simulink library "InputDeviceHandler"  (R2016b)
settings: Solver=VariableStepAuto  StartTime=0.0  StopTime=10.0  RelTol=1e-3
settings Model: Creator=Nathan  LastModifiedBy=march

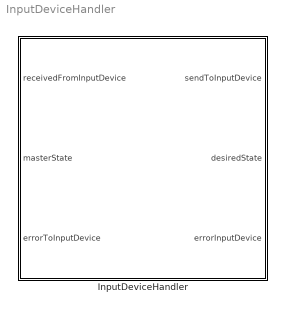
== system InputDeviceHandler ==
  InputDeviceHandler : Subsystem

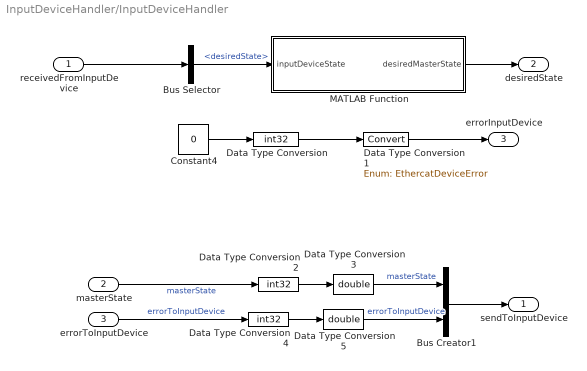
== system InputDeviceHandler/InputDeviceHandler ==
  receivedFromInputDevice : Inport  OutDataTypeStr=Bus: EtherCATReceivedFromInputDevice  BusOutputAsStruct=on
  masterState : Inport  Port=2  OutDataTypeStr=Enum: ExoskeletonState
  errorToInputDevice : Inport  Port=3
  Bus Creator1 : BusCreator  Inputs=2  OutDataTypeStr=Bus: EtherCATSendToInputDevice  NonVirtualBus=on
  Bus Selector : BusSelector  OutputSignals=desiredState
  Constant4 : Constant  Value=0
      settings: OpenFcn=|
      | b = get_param(gcb,'value');
      | if (strcmp(b,'72')),
      |   set_param (gcb,'value','0');
      | else
      |   set_param(gcb,'value','72');
      | end;
  Data Type Conversion : DataTypeConversion  OutDataTypeStr=int32
  Data Type Conversion1 : DataTypeConversion  OutDataTypeStr=Enum: EthercatDeviceError
  Data Type Conversion2 : DataTypeConversion  OutDataTypeStr=int32
  Data Type Conversion3 : DataTypeConversion  OutDataTypeStr=double
  Data Type Conversion4 : DataTypeConversion  OutDataTypeStr=int32
  Data Type Conversion5 : DataTypeConversion  OutDataTypeStr=double
  MATLAB Function : MATLAB Function  TreatAsAtomicUnit=on
  sendToInputDevice : Outport  OutDataTypeStr=Bus: EtherCATSendToInputDevice  BusOutputAsStruct=on
  desiredState : Outport  Port=2
  errorInputDevice : Outport  Port=3  OutDataTypeStr=Enum: EthercatDeviceError
  wires:
  Data Type Conversion5/1 -> Bus Creator1/2  "errorToInputDevice"
  errorToInputDevice/1 -> Data Type Conversion4/1  "errorToInputDevice"
  Data Type Conversion4/1 -> Data Type Conversion5/1
  Data Type Conversion3/1 -> Bus Creator1/1  "masterState"
  Data Type Conversion2/1 -> Data Type Conversion3/1
  MATLAB Function/1(desiredMasterState) -> desiredState/1
  Bus Selector/1 -> MATLAB Function/1(inputDeviceState)  "<desiredState>"
  receivedFromInputDevice/1 -> Bus Selector/1
  Data Type Conversion1/1 -> errorInputDevice/1
  Data Type Conversion/1 -> Data Type Conversion1/1
  masterState/1 -> Data Type Conversion2/1  "masterState"
  Bus Creator1/1 -> sendToInputDevice/1
  Constant4/1 -> Data Type Conversion/1

== matlab function InputDeviceHandler/MATLAB Function ==
  data: inputDeviceState input; desiredMasterState output
function desiredMasterState = getDesiredMasterState(inputDeviceState)
%% Translates received inputDeviceState to desired ExoskeletonState
% Copy of input device source code:
%#define SIT 0
%#define STAND 1
%#define WALK 2
%#define STONES 3
%#define STAIRS_UP 4
%#define STAIRS_DOWN 5
%#define SLOPE_UP 6
%#define SLOPE_DOWN 7
%#define MANUAL 8
switch(inputDeviceState)
    case 0 %% on disconnect, this will be zero. Need to change the values in inputDevice source
        desiredMasterState = ExoskeletonState.SITTINGDOWN;
    case 1
        desiredMasterState = ExoskeletonState.STANDINGUP;
    case 2
        desiredMasterState = ExoskeletonState.CONTINUOUSGAIT;
    case 3
        desiredMasterState = ExoskeletonState.STONES;
    case 4
        desiredMasterState = ExoskeletonState.STAIRS; %% only one stairs currently
    case 5
        desiredMasterState = ExoskeletonState.STAIRS;
    case 6
        desiredMasterState = ExoskeletonState.SLOPE; %% only one slope currently
    case 7
        desiredMasterState = ExoskeletonState.SLOPE;
    case 8
        desiredMasterState = ExoskeletonState.MANUAL;
    otherwise
        desiredMasterState = ExoskeletonState.FULLMANUAL;
end
end
